simulink model "A12_dead_beat_upravuvac_primer_3"  (R2018a)
settings: Solver=VariableStepAuto  StartTime=0.0  StopTime=20.0  RelTol=1e-3
settings Model: Creator=milam  LastModifiedBy=milam

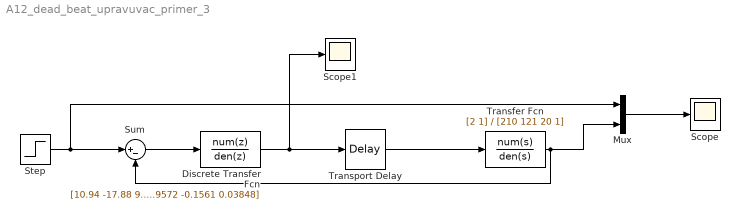
== system A12_dead_beat_upravuvac_primer_3 ==
  Discrete Transfer Fcn : DiscreteTransferFcn  Numerator=[10.94 -17.88 9.925 -2.135 0.1478]  Denominator=[1 0.07489 -0.9572 -0.1561 0.03848]  SampleTime=4
  Mux : Mux  Inputs=2
  Scope : Scope
  Scope1 : Scope
  Step : Step  Time=0  SampleTime=4
  Sum : Sum  Inputs=|+-
  Transfer Fcn : TransferFcn  Numerator=[2 1]  Denominator=[210 121 20 1]
  Transport Delay : TransportDelay  DelayTime=4
  wires:
  Step/1 -> Mux/1, Sum/1
  Sum/1 -> Discrete Transfer Fcn/1
  Discrete Transfer Fcn/1 -> Scope1/1, Transport Delay/1
  Transport Delay/1 -> Transfer Fcn/1
  Transfer Fcn/1 -> Sum/2, Mux/2
  Mux/1 -> Scope/1
